simulink model "sul_elevator_a320_main"  (R2022b)
settings: Solver=ode4  StartTime=0.0  StopTime=40  FixedStep=0.0001  RelTol=1e-3
InitFcn:
  | sul_elevator_a320_initialData
StartFcn:
  | sul_elevator_a320_initialData
values from neighbouring files (symbols this model uses):
  A_1 = 5.03*1e-3    (= 0.00503)    [sul_elevator_a320_initialData.m]
  A_2 = 1.59*1e-3    (= 0.00159)    [sul_elevator_a320_initialData.m]
  delta = -25:0.1:25    [sul_elevator_a320_initialData.m]
  delta_dyn = deg2rad(delta_dyn)    [sul_elevator_a320_initialData.m]
  delta_h = -(Y-sqrt(L^2+R^2-2*L*R*cos(alpha_prim-delta*pi/180)))    [sul_elevator_a320_initialData.m]
  K = 1.8e5    (= 180000)    [sul_elevator_a320_initialData.m]
  m = 10    [sul_elevator_a320_initialData.m]
  p_01 = 1e6    (= 1000000)    [sul_elevator_a320_initialData.m]
  p_02 = p_01*A_1/A_2    (= 3163522.01258)    [sul_elevator_a320_initialData.m]
  Q = V.^2*R_B    [sul_elevator_a320_initialData.m]
  V = (0.1*v_dzwieku:10:0.8*v_dzwieku)'    [sul_elevator_a320_initialData.m]
  V_1 = 2.26*1e-4    (= 0.000226)    [sul_elevator_a320_initialData.m]
  V_2 = 6.68*1e-5    (= 6.68e-05)    [sul_elevator_a320_initialData.m]
  v_lotu = 0.5*340    (= 170)    [sul_elevator_a320_initialData.m]
  x_0 = 0    [sul_elevator_a320_initialData.m]
  xp_0 = 0    [sul_elevator_a320_initialData.m]
libraries: slpidlib x1
settings Model: Creator=julia  LastModifiedBy=lukas

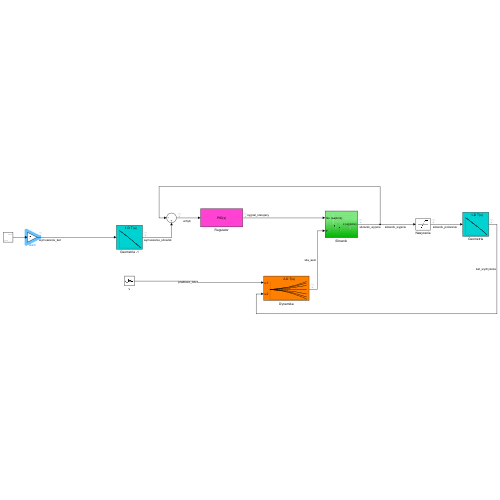
[thumbnail: Simulink's stored preview of the top-level diagram]
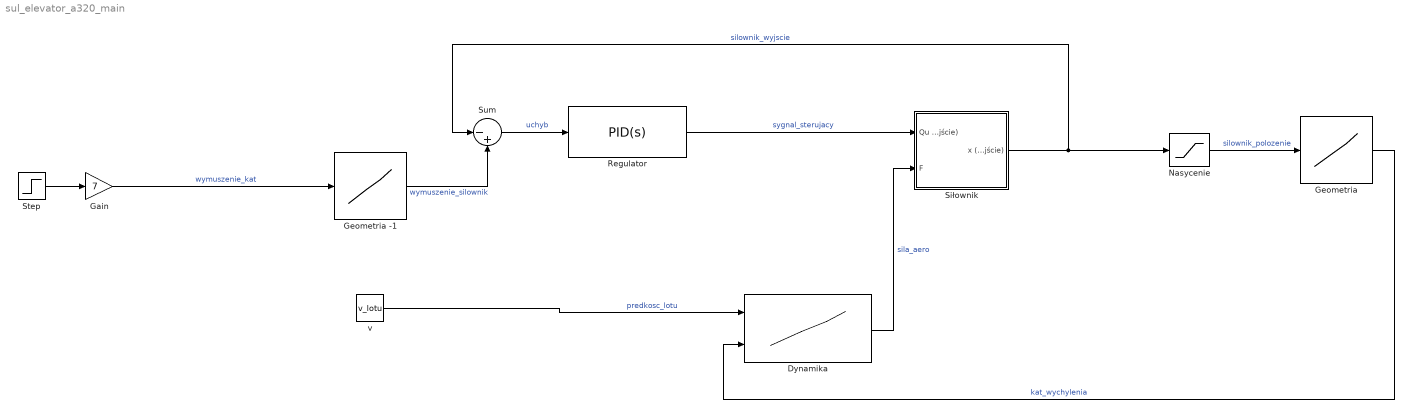
== system sul_elevator_a320_main ==
  Dynamika : Lookup_n-D  BreakpointsForDimension1=V  BreakpointsForDimension2=delta_dyn  Table=Q  InternalRulePriority=Speed  RndMeth=Simplest
      settings: InputPortMap=u0,u1
  Gain : Gain  Gain=7
  Geometria : Lookup_n-D  NumberOfTableDimensions=1  BreakpointsForDimension1=flip(delta_h)  Table=flip(delta)  InternalRulePriority=Speed  RndMeth=Simplest
  Geometria -1 : Lookup_n-D  NumberOfTableDimensions=1  BreakpointsForDimension1=delta  Table=delta_h  InternalRulePriority=Speed  RndMeth=Simplest
  Nasycenie : Saturate  UpperLimit=max(delta_h)  LowerLimit=min(delta_h)
  Regulator : slpidlib/PID Controller  Controller=PID  Form=Parallel  TimeDomain=Continuous-time  UseExternalTs=off  SampleTime=-1  IntegratorMethod=Forward Euler  FilterMethod=Forward Euler  ControllerParametersSource=internal  P=0.00799966383741104  I=0.00385710651572834  UseKiTs=off  D=-0.00120567932069365  N=6.63498469295193  UseFilter=on  TunerSelectOption=Transfer Function Based (PID Tuner App)  InitialConditionSource=internal  InitialConditionForIntegrator=0  InitialConditionForFilter=0  DifferentiatorICPrevScaledInput=0  ExternalReset=none  TrackingMode=off  Kt=1  LimitOutput=off  SatLimitsSource=internal  UpperSaturationLimit=inf  LowerSaturationLimit=-inf  LinearizeAsGain=on  AntiWindupMode=none  Kb=1  LimitIntegrator=off  UpperIntegratorSaturationLimit=inf  LowerIntegratorSaturationLimit=-inf  POutMin=[]  POutMax=[]  IOutMin=[]  IOutMax=[]  DOutMin=[]  DOutMax=[]  NOutMin=[]  NOutMax=[]  SumOutMin=[]  SumOutMax=[]  SaturationOutMin=[]  SaturationOutMax=[]  PParamMin=[]  PParamMax=[]  IParamMin=[]  IParamMax=[]  DParamMin=[]  DParamMax=[]  NParamMin=[]  NParamMax=[]  KbParamMin=[]  KbParamMax=[]  KtParamMin=[]  KtParamMax=[]  KbOutMin=[]  KbOutMax=[]  KtOutMin=[]  KtOutMax=[]  IntegratorOutMin=[]  IntegratorOutMax=[]  FilterOutMin=[]  FilterOutMax=[]  SumI1OutMin=[]  SumI1OutMax=[]  SumI2OutMin=[]  SumI2OutMax=[]  SumI3OutMin=[]  SumI3OutMax=[]  SumI4OutMin=[]  SumI4OutMax=[]  SumDOutMin=[]  SumDOutMax=[]  DifferentiatorOutMin=[]  DifferentiatorOutMax=[]  FilterDiffOutCoefMin=[]  FilterDiffOutCoefMax=[]  ReciprocalOutMin=[]  ReciprocalOutMax=[]  SumDenOutMin=[]  SumDenOutMax=[]  SumNumOutMin=[]  SumNumOutMax=[]  DivideOutMin=[]  DivideOutMax=[]  UdiffTsProdOutMin=[]  UdiffTsProdOutMax=[]  NTsProdOutMin=[]  NTsProdOutMax=[]  UintegralTsProdOutMin=[]  UintegralTsProdOutMax=[]  UngainTsProdOutMin=[]  UngainTsProdOutMax=[]  ClampingZeroOutDataTypeStr=Inherit: Inherit via back propagation  ClampingZeroOutMin=[]  ClampingZeroOutMax=[]  FilterDenConstantOutDataTypeStr=Inherit: Inherit via back propagation  FilterDenConstantOutMin=[]  FilterDenConstantOutMax=[]  PCopyOutDataTypeStr=Inherit: Inherit via back propagation  PCopyOutMin=[]  PCopyOutMax=[]  NCopyOutDataTypeStr=Inherit: Inherit via back propagation  NCopyOutMin=[]  NCopyOutMax=[]  IntegratorContinuousStateAttributes=''  IntegratorStateMustResolveToSignalObject=off  IntegratorRTWStateStorageClass=Auto  FilterContinuousStateAttributes=''  FilterStateMustResolveToSignalObject=off  FilterRTWStateStorageClass=Auto  ParallelPVariant=InternalParameters  IdealPVariant=Disabled  IVariant=InternalParameters  DVariant=InternalParameters  IntegratorVariant=Continuous  SatVariant=Disabled  AWVariant=Passthrough  PCopyVariant=Disabled  TRVariant=Disabled  FdbkBlocksVariant=Forward  IdealPFdbkVariant=Disabled  SatFdbkVariant=Disabled  DerivativeFilterVariant=ContFilter  NVariant=InternalParameters  NCopyVariant=Disabled  FilterICVariant=InternalICsFilter  IntegratorICVariant=InternalICs  ExternalResetVariant=Disabled  TRSumVariant=Passthrough  SumFdbkVariant=Disabled  SumVariant=Sum_PID  TsampFilterVariant=InternalTs  TsampNgainVariant=Passthrough  TsampIntegralVariant=Passthrough  ExternalSaturationOutDataTypeStr=Inherit: Same as second input
  Siłownik : Subsystem
  Step : Step  SampleTime=0
  Sum : Sum  Inputs=|-+
  v : Constant  Value=v_lotu
  wires:
  Geometria/1 -> Dynamika/2  "kat_wychylenia"
  Dynamika/1 -> Siłownik/2(F)  "sila_aero"
  v/1 -> Dynamika/1  "predkosc_lotu"
  Geometria -1/1 -> Sum/2  "wymuszenie_silownik"
  Sum/1 -> Regulator/1  "uchyb"
  Step/1 -> Gain/1
  Regulator/1 -> Siłownik/1(Qu (wejście))  "sygnal_sterujacy"
  Siłownik/1(x (wyjście)) -> Nasycenie/1, Sum/1  "silownik_wyjscie"
  Gain/1 -> Geometria -1/1  "wymuszenie_kat"
  Nasycenie/1 -> Geometria/1  "silownik_polozenie"

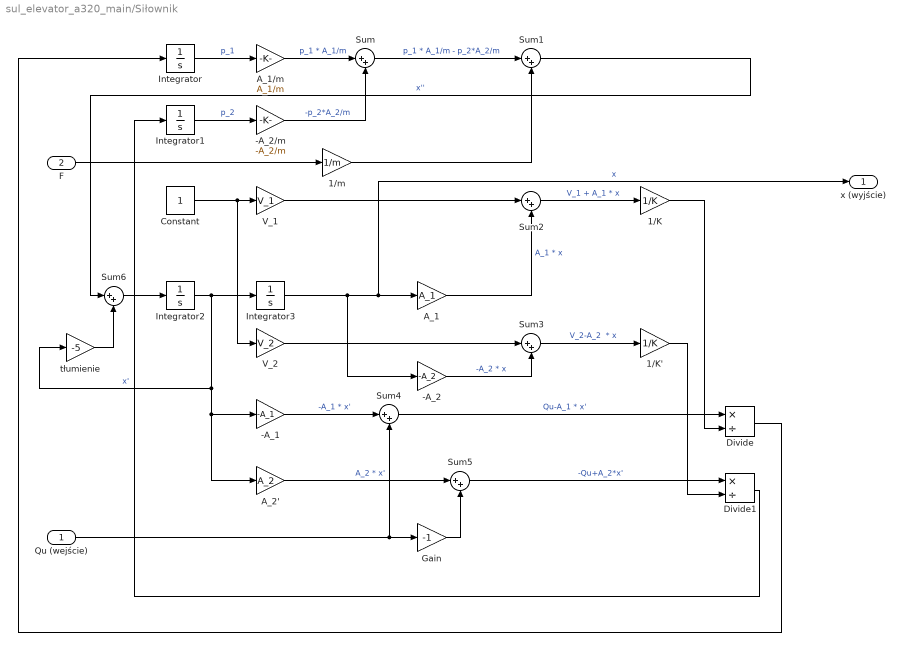
== system sul_elevator_a320_main/Siłownik ==
  Qu (wejście) : Inport
  F : Inport  Port=2
  -A_1 : Gain  Gain=-A_1
  -A_2 : Gain  Gain=-A_2
  -A_2/m : Gain  Gain=-A_2/m
  1/K : Gain  Gain=1/K
  1/K' : Gain  Gain=1/K
  1/m : Gain  Gain=1/m
  A_1 : Gain  Gain=A_1
  A_1/m : Gain  Gain=A_1/m
  A_2' : Gain  Gain=A_2
  Constant : Constant
  Divide : Product  Inputs=*/
  Divide1 : Product  Inputs=*/
  Gain : Gain  Gain=-1
  Integrator : Integrator  InitialCondition=p_01
  Integrator1 : Integrator  InitialCondition=p_02
  Integrator2 : Integrator  InitialCondition=xp_0
  Integrator3 : Integrator  InitialCondition=x_0
  Sum{,1..6} (7 alike) : Sum  Inputs=|++
  V_1 : Gain  Gain=V_1
  V_2 : Gain  Gain=V_2
  tłumienie : Gain  Gain=-5
  x (wyjście) : Outport
  wires:
  Integrator/1 -> A_1/m/1  "p_1"
  A_1/m/1 -> Sum/1  "p_1 * A_1/m"
  Integrator1/1 -> -A_2/m/1  "p_2"
  -A_2/m/1 -> Sum/2  "-p_2*A_2/m"
  Sum/1 -> Sum1/1  "p_1 * A_1/m - p_2*A_2/m"
  Integrator2/1 -> Integrator3/1, A_2'/1, -A_1/1, tłumienie/1  "x'"
  Integrator3/1 -> -A_2/1, x (wyjście)/1, A_1/1  "x"
  Constant/1 -> V_2/1, V_1/1
  V_1/1 -> Sum2/1
  A_1/1 -> Sum2/2  "A_1 * x"
  -A_2/1 -> Sum3/2  "-A_2 * x"
  V_2/1 -> Sum3/1
  Sum2/1 -> 1/K/1  "V_1 + A_1 * x"
  Sum3/1 -> 1/K'/1  "V_2-A_2  * x"
  Qu (wejście)/1 -> Gain/1, Sum4/2
  -A_1/1 -> Sum4/1  "-A_1 * x'"
  A_2'/1 -> Sum5/1  "A_2 * x'"
  Sum4/1 -> Divide/1  "Qu-A_1 * x'"
  1/K/1 -> Divide/2
  Sum5/1 -> Divide1/1  "-Qu+A_2*x'"
  1/K'/1 -> Divide1/2
  Divide/1 -> Integrator/1
  Divide1/1 -> Integrator1/1
  Gain/1 -> Sum5/2
  F/1 -> 1/m/1
  1/m/1 -> Sum1/2
  Sum1/1 -> Sum6/1  "x''"
  tłumienie/1 -> Sum6/2
  Sum6/1 -> Integrator2/1
